simulink model "c1ex4mod"  (Simulink 5.1)
settings: Solver=ode45  StartTime=0.0  StopTime=1200.0  RelTol=1e-6
settings Model: LastModifiedBy=hc  BooleanDataType=on  ProdHWDeviceType=Microprocessor

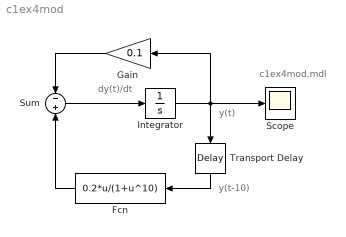
== system c1ex4mod ==
  note: y(t)
  note: y(t-10)
  note: dy(t)/dt
  note: c1ex4mod.mdl
  Fcn : Fcn  Orientation=left  Expr=0.2*u/(1+u^10)
  Gain : Gain  Orientation=left  Gain=0.1  SaturateOnIntegerOverflow=on
  Integrator : Integrator  InitialCondition=0.1
  Scope : Scope
      settings: TimeRange=1200  YMin=-0.2678571428571441  YMax=1.81547619047619
  Sum : Sum  Inputs=-|+  SaturateOnIntegerOverflow=on  InputSameDT=on
  Transport Delay : TransportDelay  Orientation=down  DelayTime=30
  wires:
  Integrator/1 -> Transport Delay/1, Gain/1, Scope/1
  Transport Delay/1 -> Fcn/1
  Sum/1 -> Integrator/1
  Fcn/1 -> Sum/2
  Gain/1 -> Sum/1
